simulink model "modello_non_lineare"  (R2022b)
settings: Solver=VariableStepAuto  StartTime=0.0  StopTime=10.0  RelTol=1e-3
model workspace (MAT data in the model file):
  omegaValue = Simulink.Parameter
  omegaValue.Value = 90
  omegaValue.DataType = 'auto'
  omegaValue.Complexity = 'real'
  omegaValue.Dimensions = [1 1]
  thetaValue = Simulink.Parameter
  thetaValue.Value = 0
  thetaValue.DataType = 'auto'
  thetaValue.Complexity = 'real'
  thetaValue.Dimensions = [1 1]
settings Model: ParameterArgumentNames=omegaValue,thetaValue  Creator=eleon  LastModifiedBy=eleon

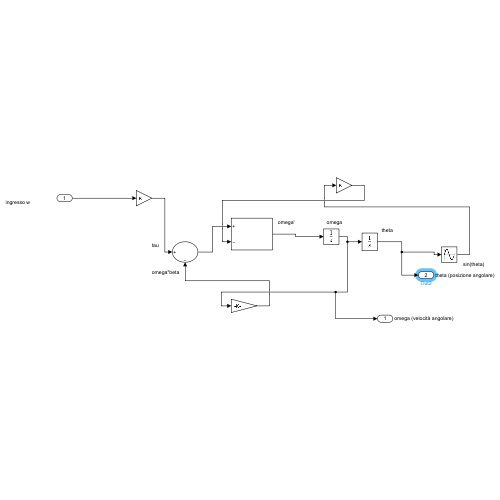
[thumbnail: Simulink's stored preview of the top-level diagram]
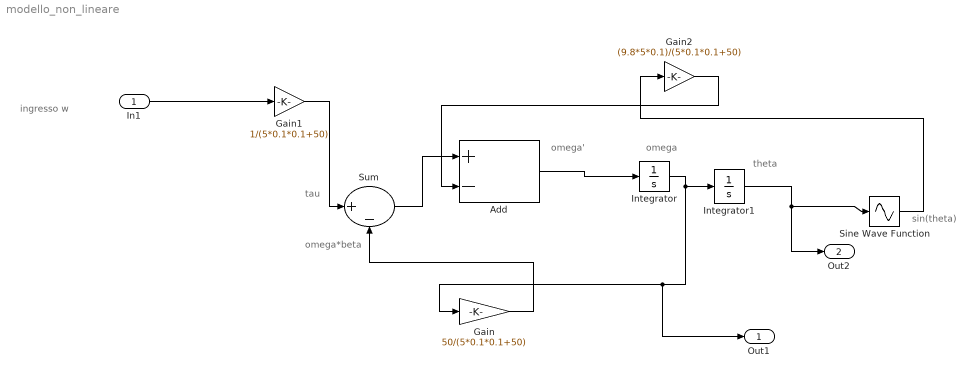
== system modello_non_lineare ==
  note: omega'
  note: tau
  note: theta
  note: ingresso w
  note: omega
  note: sin(theta)
  note: omega*beta
  In1 : Inport
  Add : Sum  Inputs=+-
  Gain : Gain  Gain=50/(5*0.1*0.1+50)
  Gain1 : Gain  Gain=1/(5*0.1*0.1+50)
  Gain2 : Gain  Gain=(9.8*5*0.1)/(5*0.1*0.1+50)
  Integrator : Integrator  InitialCondition=omegaValue  mask{omega=omegaValue}
      mask prompts: omega "Velocità omega"
  Integrator1 : Integrator  InitialCondition=theta  mask{theta=thetaValue}
      mask prompts: theta "Angolo theta"
  Sine Wave Function : Sin  TimeSource=Use external signal  SampleTime=0
  Sum : Sum  Inputs=|+-
  Out1 : Outport  SignalName=omega (velocità angolare)
  Out2 : Outport  Port=2  SignalName=theta (posizione angolare)
  wires:
  Integrator1/1 -> Out2/1, Sine Wave Function/1
  Gain1/1 -> Sum/1
  Gain2/1 -> Add/2
  Add/1 -> Integrator/1
  Gain/1 -> Sum/2
  Sine Wave Function/1 -> Gain2/1
  Sum/1 -> Add/1
  Integrator/1 -> Out1/1, Gain/1, Integrator1/1
  In1/1 -> Gain1/1
